simulink model "Conference2"  (R2019b)
settings: Solver=ode23tb  StartTime=0.0  StopTime=10.0  RelTol=1e-3
libraries: powerlib x43, simulink x1
settings Model: Creator=jarir  LastModifiedBy=jarir
settings SolverCC: MaxOrder=2

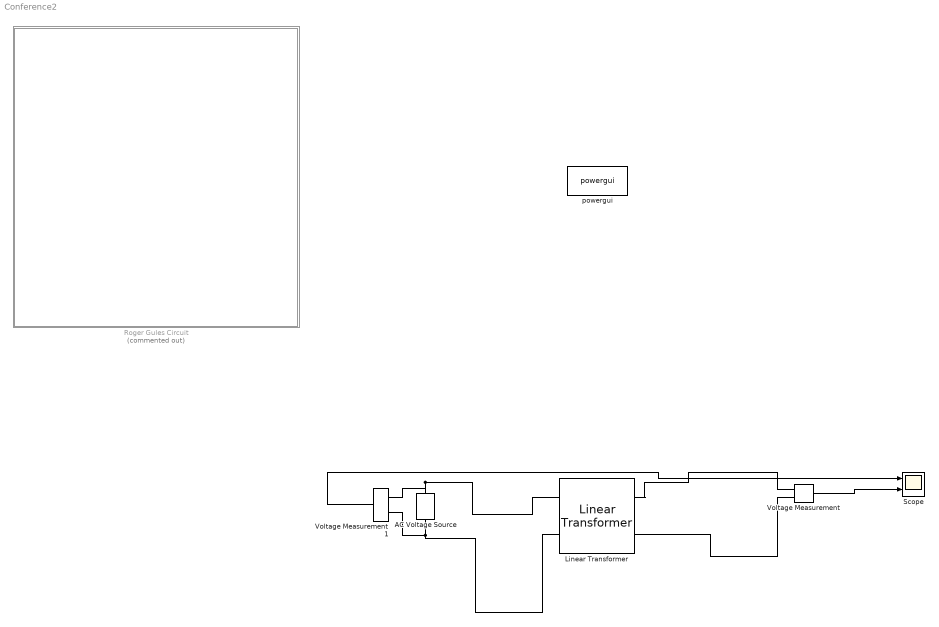
== system Conference2 ==
  AC Voltage Source : powerlib/Electrical Sources/AC Voltage Source  Amplitude=325  Phase=0  Frequency=50  SampleTime=0  Measurements=None  BusType=swing  Pref=10e3  Qref=0  Qmin=-inf  Qmax=+inf
      settings: SourceProductName=Simscape Electrical
  Linear Transformer : powerlib/Elements/Linear Transformer  UNITS=pu  NominalPower=[ 250e6 60 ]  winding1="[ 735e3  0.002  0.08 ]"  winding2="[ 315e3  0.002  0.08 ]"  ThreeWindings=off  winding3=[ 315e3 0.002 0.08 ]  RmLm=[ 500 500 ]  Measurements=None  DataType=off
      settings: SourceProductName=Simscape Electrical
  Roger Gules Circuit : Subsystem  Commented=on
  Scope : Scope  NumInputPorts=2
  Voltage Measurement : powerlib/Measurements/Voltage Measurement  PhasorSimulation=off  OutputType=Complex  PSBequivalent=0
      settings: SourceProductName=Simscape Electrical
  Voltage Measurement1 : powerlib/Measurements/Voltage Measurement  PhasorSimulation=off  OutputType=Complex  PSBequivalent=0
      settings: SourceProductName=Simscape Electrical
  powergui : powerlib/powergui  Priority=1  SimulationMode=Continuous  SampleTime=50e-6  frequency=60  Iterations=50  frequencyindice=50  Pbase=100e6  ErrMax=1e-4  UnitsV=kV  UnitsW=MW  buscounter=0  FunctionMessages=off  echomessages=off  EnableUseOfTLC=off  CurrentSourceSwitches=off  DisableSnubberDevices=off  DisableRonSwitches=off  DisableVfSwitches=off  DisplayEquations=off  AutomaticDiscreteSolvers=off  SolverType=Tustin/Backward Euler (TBE)  Interpol=off  ExternalGateDelay=off  methode=off  Ts=100  x0status=blocks  SPID=on  SwTol=0  HookPort=off  NonlinearTolerance=1e-4  nMaxIteration=100  ContinueOnMaxIteration=off  RestoreLinks=warning  ResistiveCurrentMeasurement=off  Frange=[0:2:500]  Ylog=off  Xlog=on  ShowGrid=off  save=off  variable=ZData  structure=0  ZoomFFT=off  StartTime=0.0  cycles=1  DisplayStyle=1  fundamental=60  FreqAxis=off  MaxFrequency=1000  frequencyindicesteady=1  RmsSteady=1  display=off
      settings: SourceProductName=Simscape Electrical
  wires:
  Voltage Measurement/1 -> Scope/2
  Voltage Measurement1/1 -> Scope/1
  connections:
  AC Voltage Source/RConn1 -- Linear Transformer/LConn1 -- Voltage Measurement1/LConn1
  Voltage Measurement1/LConn2 -- Linear Transformer/LConn2 -- AC Voltage Source/LConn1
  Linear Transformer/RConn1 -- Voltage Measurement/LConn1
  Voltage Measurement/LConn2 -- Linear Transformer/RConn2

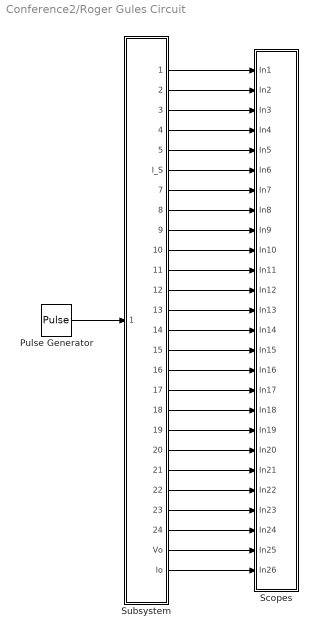
== system Conference2/Roger Gules Circuit ==
  Pulse Generator : DiscretePulseGenerator  PulseType=Time based  Period=1/50000  PulseWidth=75
  Scopes : Subsystem
  Subsystem : Subsystem
  wires:
  Subsystem/9(V_Dm1) -> Scopes/9(In9)
  Subsystem/8(I_CS1) -> Scopes/8(In8)
  Subsystem/18(I_Dm2) -> Scopes/18(In18)
  Subsystem/1(V_in) -> Scopes/1(In1)
  Subsystem/3(V_L1) -> Scopes/3(In3)
  Subsystem/24(I_Co) -> Scopes/24(In24)
  Subsystem/13(V_L2s) -> Scopes/13(In13)
  Subsystem/7(V_Cs1) -> Scopes/7(In7)
  Subsystem/2(I_in) -> Scopes/2(In2)
  Subsystem/10(I_Dm1) -> Scopes/10(In10)
  Subsystem/6(I_S) -> Scopes/6(In6)
  Subsystem/23(V_Co) -> Scopes/23(In23)
  Subsystem/12(I_L2p) -> Scopes/12(In12)
  Subsystem/14(I_L2s) -> Scopes/14(In14)
  Subsystem/15(V_Cs2) -> Scopes/15(In15)
  Subsystem/11(V_L2p) -> Scopes/11(In11)
  Subsystem/17(V_Dm2) -> Scopes/17(In17)
  Subsystem/19(V_Cm) -> Scopes/19(In19)
  Subsystem/26(Io) -> Scopes/26(In26)
  Subsystem/21(V_Do) -> Scopes/21(In21)
  Subsystem/20(I_Cm) -> Scopes/20(In20)
  Subsystem/5(V_S) -> Scopes/5(In5)
  Subsystem/16(I_CS2) -> Scopes/16(In16)
  Subsystem/25(Vo) -> Scopes/25(In25)
  Subsystem/22(I_Do) -> Scopes/22(In22)
  Pulse Generator/1 -> Subsystem/1(In1)
  Subsystem/4(I_L1) -> Scopes/4(In4)

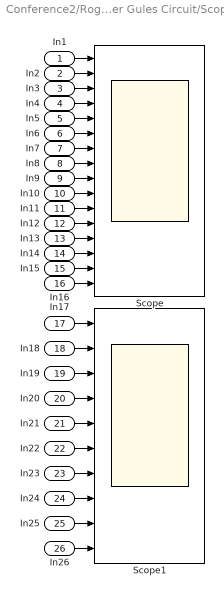
== system Conference2/Roger Gules Circuit/Scopes ==
  In1 : Inport
  In2 : Inport  Port=2
  In3 : Inport  Port=3
  In4 : Inport  Port=4
  In5 : Inport  Port=5
  In6 : Inport  Port=6
  In7 : Inport  Port=7
  In8 : Inport  Port=8
  In9 : Inport  Port=9
  In10 : Inport  Port=10
  In11 : Inport  Port=11
  In12 : Inport  Port=12
  In13 : Inport  Port=13
  In14 : Inport  Port=14
  In15 : Inport  Port=15
  In16 : Inport  Port=16
  In17 : Inport  Port=17
  In18 : Inport  Port=18
  In19 : Inport  Port=19
  In20 : Inport  Port=20
  In21 : Inport  Port=21
  In22 : Inport  Port=22
  In23 : Inport  Port=23
  In24 : Inport  Port=24
  In25 : Inport  Port=25
  In26 : Inport  Port=26
  Scope : Scope  NumInputPorts=16
  Scope1 : Scope  NumInputPorts=10
  wires:
  In22/1 -> Scope1/6
  In23/1 -> Scope1/7
  In1/1 -> Scope/1
  In7/1 -> Scope/7
  In26/1 -> Scope1/10
  In2/1 -> Scope/2
  In25/1 -> Scope1/9
  In24/1 -> Scope1/8
  In5/1 -> Scope/5
  In9/1 -> Scope/9
  In13/1 -> Scope/13
  In3/1 -> Scope/3
  In11/1 -> Scope/11
  In17/1 -> Scope1/1
  In18/1 -> Scope1/2
  In21/1 -> Scope1/5
  In16/1 -> Scope/16
  In19/1 -> Scope1/3
  In20/1 -> Scope1/4
  In8/1 -> Scope/8
  In10/1 -> Scope/10
  In15/1 -> Scope/15
  In12/1 -> Scope/12
  In6/1 -> Scope/6
  In14/1 -> Scope/14
  In4/1 -> Scope/4

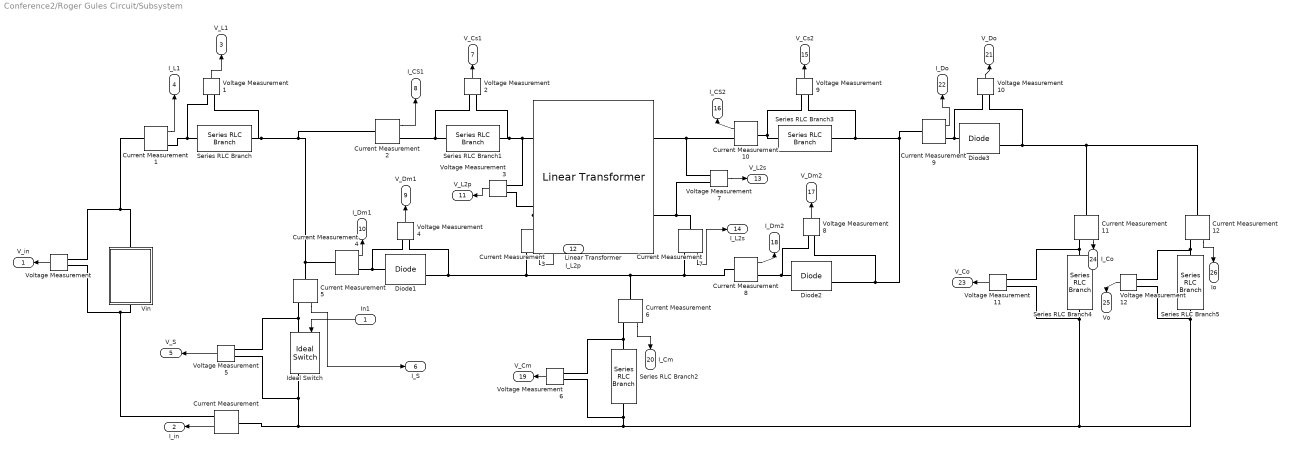
== system Conference2/Roger Gules Circuit/Subsystem ==
  In1 : Inport
  Current Measurement{,1..12} (13 alike) : powerlib/Measurements/Current Measurement  PhasorSimulation=off  OutputType=Complex  PSBequivalent=0
      settings: SourceProductName=Simscape Electrical
  Diode1 : powerlib/Power Electronics/Diode  Ron=0.001  Lon=0  Vf=0.8  IC=0  UseSnubber=0  Rs=500  Cs=250e-9  Measurements=on
      settings: SourceProductName=Simscape Electrical
  Diode2 : powerlib/Power Electronics/Diode  Ron=0.001  Lon=0  Vf=0.8  IC=0  UseSnubber=0  Rs=500  Cs=250e-9  Measurements=on
      settings: SourceProductName=Simscape Electrical
  Diode3 : powerlib/Power Electronics/Diode  Ron=0.001  Lon=0  Vf=0.8  IC=0  UseSnubber=0  Rs=500  Cs=250e-9  Measurements=on
      settings: SourceProductName=Simscape Electrical
  Ideal Switch : powerlib/Power Electronics/Ideal Switch  Ron=0.001  Lon=0  IC=0  Rs=1e5  Cs=inf  Measurements=on
      settings: SourceProductName=Simscape Electrical
  Linear Transformer : powerlib/Elements/Linear Transformer  UNITS=pu  NominalPower=[ 250e6 50e3 ]  winding1="[ 735e3  0  0 ]"  winding2="[ 315e3  0  0 ]"  ThreeWindings=off  winding3=[ 315e3 0.002 0.08 ]  RmLm=[ inf inf ]  Measurements=None  DataType=off
      settings: SourceProductName=Simscape Electrical
  Series RLC Branch : powerlib/Elements/Series RLC Branch  LConnTagsString=__new0  RConnTagsString=__new0  BranchType=L  Resistance=1  Inductance=220e-6  SetiL0=off  InitialCurrent=0  Capacitance=1e-6  Setx0=off  InitialVoltage=0  Measurements=None
      settings: SourceProductName=Simscape Electrical
  Series RLC Branch{1..4} (4 alike) : powerlib/Elements/Series RLC Branch  LConnTagsString=__new0  RConnTagsString=__new0  BranchType=C  Resistance=1  Inductance=220e-6  SetiL0=off  InitialCurrent=0  Capacitance=220e-6  Setx0=off  InitialVoltage=0  Measurements=None
      settings: SourceProductName=Simscape Electrical
  Series RLC Branch5 : powerlib/Elements/Series RLC Branch  LConnTagsString=__new0  RConnTagsString=__new0  BranchType=R  Resistance=320  Inductance=220e-6  SetiL0=off  InitialCurrent=0  Capacitance=220e-6  Setx0=off  InitialVoltage=0  Measurements=None
      settings: SourceProductName=Simscape Electrical
  Vin : Subsystem
  Voltage Measurement{,1..12} (13 alike) : powerlib/Measurements/Voltage Measurement  PhasorSimulation=off  OutputType=Complex  PSBequivalent=0
      settings: SourceProductName=Simscape Electrical
  V_in : Outport
  I_in : Outport  Port=2
  V_L1 : Outport  Port=3
  I_L1 : Outport  Port=4
  V_S : Outport  Port=5
  I_S : Outport  Port=6
  V_Cs1 : Outport  Port=7
  I_CS1 : Outport  Port=8
  V_Dm1 : Outport  Port=9
  I_Dm1 : Outport  Port=10
  V_L2p : Outport  Port=11
  I_L2p : Outport  Port=12
  V_L2s : Outport  Port=13
  I_L2s : Outport  Port=14
  V_Cs2 : Outport  Port=15
  I_CS2 : Outport  Port=16
  V_Dm2 : Outport  Port=17
  I_Dm2 : Outport  Port=18
  V_Cm : Outport  Port=19
  I_Cm : Outport  Port=20
  V_Do : Outport  Port=21
  I_Do : Outport  Port=22
  V_Co : Outport  Port=23
  I_Co : Outport  Port=24
  Vo : Outport  Port=25
  Io : Outport  Port=26
  wires:
  In1/1 -> Ideal Switch/1
  Voltage Measurement/1 -> V_in/1
  Current Measurement/1 -> I_in/1
  Voltage Measurement1/1 -> V_L1/1
  Current Measurement1/1 -> I_L1/1
  Voltage Measurement5/1 -> V_S/1
  Current Measurement5/1 -> I_S/1
  Voltage Measurement2/1 -> V_Cs1/1
  Current Measurement2/1 -> I_CS1/1
  Voltage Measurement4/1 -> V_Dm1/1
  Current Measurement4/1 -> I_Dm1/1
  Voltage Measurement3/1 -> V_L2p/1
  Current Measurement3/1 -> I_L2p/1
  Voltage Measurement7/1 -> V_L2s/1
  Current Measurement7/1 -> I_L2s/1
  Voltage Measurement9/1 -> V_Cs2/1
  Current Measurement10/1 -> I_CS2/1
  Voltage Measurement8/1 -> V_Dm2/1
  Current Measurement8/1 -> I_Dm2/1
  Voltage Measurement6/1 -> V_Cm/1
  Current Measurement6/1 -> I_Cm/1
  Voltage Measurement10/1 -> V_Do/1
  Current Measurement9/1 -> I_Do/1
  Voltage Measurement11/1 -> V_Co/1
  Current Measurement11/1 -> I_Co/1
  Voltage Measurement12/1 -> Vo/1
  Current Measurement12/1 -> Io/1
  connections:
  Current Measurement12/RConn1 -- Voltage Measurement12/LConn1 -- Series RLC Branch5/LConn1
  Current Measurement7/LConn1 -- Voltage Measurement7/LConn2 -- Linear Transformer/RConn2
  Diode1/RConn1 -- Voltage Measurement4/LConn2 -- Current Measurement7/RConn1 -- Current Measurement8/LConn1 -- Current Measurement6/LConn1 -- Current Measurement3/RConn1
  Voltage Measurement5/LConn1 -- Current Measurement5/RConn1 -- Ideal Switch/LConn1
  Current Measurement10/LConn1 -- Voltage Measurement9/LConn2 -- Series RLC Branch3/RConn1
  Current Measurement6/RConn1 -- Voltage Measurement6/LConn1 -- Series RLC Branch2/LConn1
  Current Measurement8/RConn1 -- Voltage Measurement8/LConn1 -- Diode2/LConn1
  Series RLC Branch4/LConn1 -- Voltage Measurement11/LConn1 -- Current Measurement11/RConn1
  Voltage Measurement/LConn2 -- Vin/LConn1 -- Current Measurement/RConn1
  Series RLC Branch2/RConn1 -- Voltage Measurement6/LConn2 -- Current Measurement/LConn1 -- Voltage Measurement5/LConn2 -- Ideal Switch/RConn1 -- Voltage Measurement12/LConn2 -- Series RLC Branch5/RConn1 -- Voltage Measurement11/LConn2 -- Series RLC Branch4/RConn1
  Voltage Measurement7/LConn1 -- Current Measurement10/RConn1 -- Linear Transformer/RConn1
  Current Measurement4/RConn1 -- Voltage Measurement4/LConn1 -- Diode1/LConn1
  Series RLC Branch/RConn1 -- Voltage Measurement1/LConn2 -- Current Measurement2/LConn1 -- Current Measurement5/LConn1 -- Current Measurement4/LConn1
  Series RLC Branch/LConn1 -- Current Measurement1/RConn1 -- Voltage Measurement1/LConn1
  Voltage Measurement10/LConn2 -- Current Measurement12/LConn1 -- Current Measurement11/LConn1 -- Diode3/RConn1
  Series RLC Branch1/LConn1 -- Current Measurement2/RConn1 -- Voltage Measurement2/LConn1
  Current Measurement3/LConn1 -- Voltage Measurement3/LConn2 -- Linear Transformer/LConn2
  Voltage Measurement/LConn1 -- Vin/RConn1 -- Current Measurement1/LConn1
  Current Measurement9/RConn1 -- Diode3/LConn1 -- Voltage Measurement10/LConn1
  Diode2/RConn1 -- Voltage Measurement8/LConn2 -- Current Measurement9/LConn1 -- Voltage Measurement9/LConn1 -- Series RLC Branch3/LConn1
  Linear Transformer/LConn1 -- Voltage Measurement3/LConn1 -- Voltage Measurement2/LConn2 -- Series RLC Branch1/RConn1

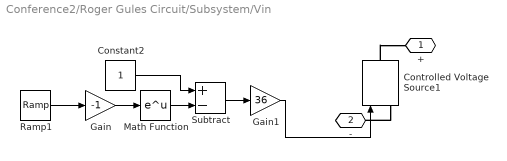
== system Conference2/Roger Gules Circuit/Subsystem/Vin ==
  Constant2 : Constant
  Controlled Voltage Source1 : powerlib/Electrical Sources/Controlled Voltage Source  Initialize=on  Source_Type=AC  Amplitude=0  Phase=0  Frequency=0  Measurements=None
      settings: SourceProductName=Simscape Electrical
  Gain : Gain  Gain=-1
  Gain1 : Gain  Gain=36
  Math Function : Math  SignedPower=off  SaturateOnIntegerOverflow=on
  Ramp1 : simulink/Sources/Ramp  slope=10  start=0  InitialOutput=0
  Subtract : Sum  Inputs=+-
  + : PMIOPort  Side=Right
  - : PMIOPort  Port=2  Side=Left
  wires:
  Gain1/1 -> Controlled Voltage Source1/1
  Constant2/1 -> Subtract/1
  Ramp1/1 -> Gain/1
  Math Function/1 -> Subtract/2
  Subtract/1 -> Gain1/1
  Gain/1 -> Math Function/1
  connections:
  Controlled Voltage Source1/RConn1 -- +/RConn1
  Controlled Voltage Source1/LConn1 -- -/RConn1
